simulink model "North_Country_Grid"  (R2025a)
settings: Solver=VariableStepAuto  StartTime=0.0  StopTime=10  RelTol=1e-3
PreLoadFcn:
  | Ts=50e-6;
InitFcn:
  | xInitial = WindFarmType4AverageModelInit;
  | Ts=50e-6;
undefined symbols (not defined in the file): D1, D11, Delta, DiscIntNeverNeededParam, find_system, Fnom_I, Fnom_R, Idc_nom, lagging, level, pulse, test_alpha, Vdc_nom, VLL_nom_I, VLL_nom_R
libraries: spsSecondOrderFilterLib x47, powerlib_extras x38, simulink x34, spsThreePhaseVIMeasurementLib x30, spsFirstOrderFilterLib x29, simulink_extras x26, spsabctodq0Lib x25, spsThreePhaseTransformerTwoWindingsLib x19, spsThreePhaseBreakerLib x18, spsThreePhasePISectionLineLib x17, spsControlledVoltageSourceLib x15, spsOnDelayLib x12
(part 10 of 18)

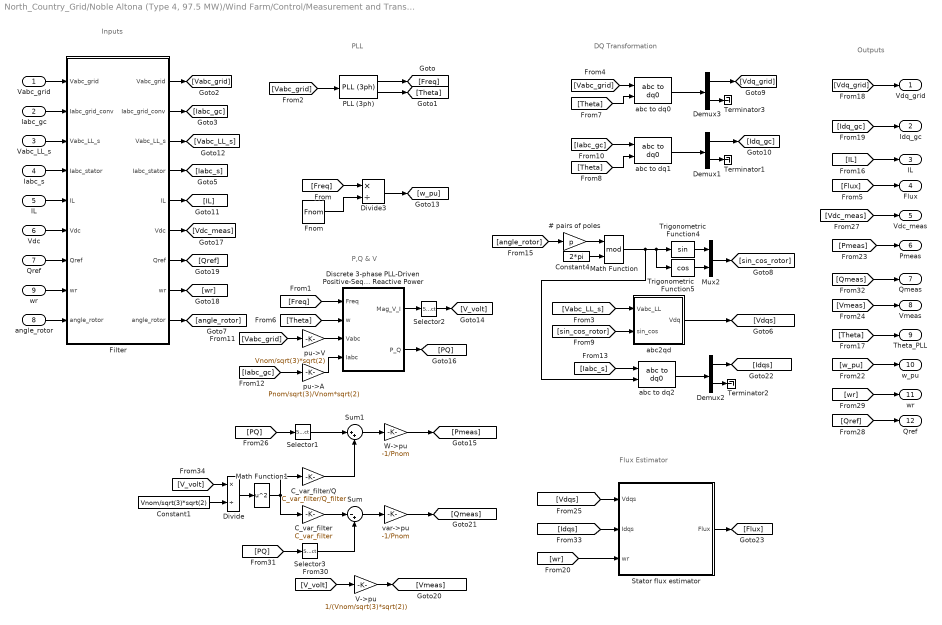
== system North_Country_Grid/Noble Altona (Type 4, 97.5 MW)/Wind Farm/Control/Measurement and Transformation ==
  note: Flux Estimator
  note: Outputs
  note: PLL
  note: DQ Transformation
  note: P,Q & V
  note: Inputs
  Vabc_grid : Inport
  Iabc_gc : Inport  Port=2
  Vabc_LL_s : Inport  Port=3
  Iabc_s : Inport  Port=4
  IL : Inport  Port=5
  Vdc : Inport  Port=6
  Qref : Inport  Port=7
  angle_rotor : Inport  Port=8
  wr : Inport  Port=9
  # pairs of poles : Gain  Gain=p  SaturateOnIntegerOverflow=on  OutDataTypeStr=Inherit: Same as input  ParamDataTypeStr=Inherit: Same as input
  C_var_filter : Gain  Gain=C_var_filter  SaturateOnIntegerOverflow=on  OutDataTypeStr=Inherit: Same as input  ParamDataTypeStr=Inherit: Same as input
  C_var_filter/Q : Gain  Gain=C_var_filter/Q_filter  SaturateOnIntegerOverflow=on  OutDataTypeStr=Inherit: Same as input  ParamDataTypeStr=Inherit: Same as input
  Constant1 : Constant  Value=Vnom/sqrt(3)*sqrt(2)
  Constant4 : Constant  Value=2*pi
  Demux1 : Demux  Outputs=[2 1]
      settings: DisplayOption=none
  Demux2 : Demux  Outputs=[2 1]
      settings: DisplayOption=none
  Demux3 : Demux  Outputs=[2 1]
      settings: DisplayOption=none
  Discrete 3-phase PLL-Driven Positive-Sequence Active & Reactive Power : Subsystem  mask(Discrete 3-phase PLL-Driven Positive-Sequence Active & Reactive Power){Finit=Fnom, Fmin=Fnom*45/60, Par_Vinit=[Vnom/sqrt(3)*sqrt(2) 30], Par_Iinit=[Pnom/sqrt(3)/Vnom*sqrt(2) -10], Ts=Ts}
      mask prompts: Finit "Initial frequency (Hz):"; Fmin "Minimum frequency (Hz):"; Par_Vinit "Voltage initial input: [ Mag  Phase(Degrees) ]"; Par_Iinit "Current initial input: [ Mag  Phase(Degrees) ]"; Ts "Sample time:"
      mask help:
      | This discrete block measures the 3-phase active power P and reactive power Q  associated with a periodic set of 3-phase voltages and currents which may contain harmonics. P and Q are calculated by evaluating the fundamental values (positive-sequence) of the input voltages and currents with a running window over one cycle of the specified frequency (port Freq).
      |  Input port "Sin_Cos" (a two-dimension signal) provides the reference frame required for the computation.
      |
      | input 1: must give the frequency of the fundamental (Hz)
      | Input 2: must contain a  [sin(wt)  cos(wt)] two dimension signal , where w is the rotation speed (rad/s) of the reference frame used for the computation..
      | input 3: Vectorized 3-phase  instantaneous voltage (Vabc)
      | input 4: Vectorized 3-phase instantaneous current (Iabc)
      |
      | Output 1: Vector [Mag_V Mag_I] of the fundamental values (Magnitude) of the voltage & current (peak values of the positive-sequence)
      | Output 2: 3-phase PQ measurement vector [P(W) Q (var)] evaluated at the specified frequency. Current flowing into an RL circuit will produce  positive active and reactive powers.
      |
      | For the first cycle of simulation, the outputs are held constant using the values specified by the parameters "Initial input".
      | he value of the parameter "Minimum frequency" is used to determine the buffer size of the "Variable Transport Delay" block found inside this subsystem.
      mask init:
      | power_initmask();
      settings: OpenFcn=power_openblockproxy();
  Divide : Product  Inputs=*/
  Divide3 : Product  Inputs=*/
  Filter : Subsystem  mask{Freq=Freq_filter, Zeta=Zeta_filter, Ts=Ts}
      mask prompts: Freq "Cut-off frequency (Hz):"; Zeta "Damping factor Zeta:"; Ts "Sample time"
  Fnom : Constant  Value=Fnom
  Math Function : Math  Operator=mod  SignedPower=on
  Math Function1 : Math  Operator=square  SignedPower=on
  Mux2 : Mux  Inputs=2
  PLL (3ph) : spsPLL3phLib/PLL (3ph)  Fmin=0.75*Fnom  Par_Init=[-45 Fnom]  ParK=[60 1400 1]  TcD=1e-4  MaxRateChangeFreq=12  FilterCutOffFreq=25  Ts=Ts  AGC=on
  Selector1 : Selector  InputPortWidth=2  IndexOptions=Index vector (dialog)  Indices=1  OutputSizes=1
  Selector2 : Selector  InputPortWidth=2  IndexOptions=Index vector (dialog)  Indices=1  OutputSizes=1
  Selector3 : Selector  InputPortWidth=2  IndexOptions=Index vector (dialog)  Indices=2  OutputSizes=1
  Stator flux estimator : Subsystem
  Sum : Sum  Inputs=|-+
  Sum1 : Sum  Inputs=|++
  Terminator1 : Terminator
  Terminator2 : Terminator
  Terminator3 : Terminator
  Trigonometric Function4 : Trigonometry
  Trigonometric Function5 : Trigonometry  Operator=cos
  V->pu : Gain  Gain=1/(Vnom/sqrt(3)*sqrt(2))  SaturateOnIntegerOverflow=on  OutDataTypeStr=Inherit: Same as input  ParamDataTypeStr=Inherit: Same as input
  W->pu : Gain  Gain=-1/Pnom  SaturateOnIntegerOverflow=on  OutDataTypeStr=Inherit: Same as input  ParamDataTypeStr=Inherit: Same as input
  abc to dq0 : spsabctodq0Lib/abc to dq0  Alignment=90 degrees behind phase A axis
  abc to dq1 : spsabctodq0Lib/abc to dq0  Alignment=90 degrees behind phase A axis
  abc to dq2 : spsabctodq0Lib/abc to dq0  Alignment=90 degrees behind phase A axis
  abc2qd : Subsystem
  pu->A : Gain  Gain=Pnom/sqrt(3)/Vnom*sqrt(2)  SaturateOnIntegerOverflow=on  OutDataTypeStr=Inherit: Same as input  ParamDataTypeStr=Inherit: Same as input
  pu->V : Gain  Gain=Vnom/sqrt(3)*sqrt(2)  SaturateOnIntegerOverflow=on  OutDataTypeStr=Inherit: Same as input  ParamDataTypeStr=Inherit: Same as input
  "var->pu " : Gain  Gain=-1/Pnom  SaturateOnIntegerOverflow=on  OutDataTypeStr=Inherit: Same as input  ParamDataTypeStr=Inherit: Same as input
  Vdq_grid : Outport  VectorParamsAs1DForOutWhenUnconnected=off
  Idq_gc : Outport  Port=2  VectorParamsAs1DForOutWhenUnconnected=off
  "IL " : Outport  Port=3  VectorParamsAs1DForOutWhenUnconnected=off
  Flux : Outport  Port=4  VectorParamsAs1DForOutWhenUnconnected=off
  Vdc_meas : Outport  Port=5  VectorParamsAs1DForOutWhenUnconnected=off
  Pmeas : Outport  Port=6  VectorParamsAs1DForOutWhenUnconnected=off
  Qmeas : Outport  Port=7  VectorParamsAs1DForOutWhenUnconnected=off
  Vmeas : Outport  Port=8  VectorParamsAs1DForOutWhenUnconnected=off
  Theta_PLL : Outport  Port=9  VectorParamsAs1DForOutWhenUnconnected=off
  w_pu : Outport  Port=10  VectorParamsAs1DForOutWhenUnconnected=off
  "wr " : Outport  Port=11  VectorParamsAs1DForOutWhenUnconnected=off
  "Qref " : Outport  Port=12  VectorParamsAs1DForOutWhenUnconnected=off
  wires:
  Filter/9("angle_rotor ") -> [angle_rotor]
  angle_rotor/1 -> Filter/9(angle_rotor)
  Stator flux estimator/1(Flux) -> [Flux]
  # pairs of poles/1 -> Math Function/1
  Constant4/1 -> Math Function/2
  abc2qd/1(Vdq) -> [Vdqs]
  Trigonometric Function5/1 -> Mux2/2
  Trigonometric Function4/1 -> Mux2/1
  [angle_rotor] -> # pairs of poles/1
  [Vabc_LL_s] -> abc2qd/1(Vabc_LL)
  [sin_cos_rotor] -> abc2qd/2(sin_cos)
  Mux2/1 -> [sin_cos_rotor]
  Demux2/1 -> [Idqs]
  Demux2/2 -> Terminator2/1
  abc to dq2/1 -> Demux2/1
  [Iabc_s] -> abc to dq2/1
  [Vdqs] -> Stator flux estimator/1(Vdqs)
  [Idqs] -> Stator flux estimator/2(Idqs)
  [wr] -> Stator flux estimator/3(wr)
  [Qmeas] -> Qmeas/1
  "var->pu "/1 -> [Qmeas]
  [PQ] -> Selector3/1
  V->pu/1 -> [Vmeas]
  [V_volt] -> V->pu/1
  Selector2/1 -> [V_volt]
  Discrete 3-phase PLL-Driven Positive-Sequence Active & Reactive Power/1(Mag_V_I) -> Selector2/1
  Demux1/2 -> Terminator1/1
  Demux3/1 -> [Vdq_grid]
  Demux3/2 -> Terminator3/1
  abc to dq1/1 -> Demux1/1
  abc to dq0/1 -> Demux3/1
  PLL (3ph)/1 -> [Freq]
  Fnom/1 -> Divide3/2
  Divide3/1 -> [w_pu]
  pu->V/1 -> Discrete 3-phase PLL-Driven Positive-Sequence Active & Reactive Power/3(Vabc)
  W->pu/1 -> [Pmeas]
  [Freq] -> Divide3/1
  [Freq] -> Discrete 3-phase PLL-Driven Positive-Sequence Active & Reactive Power/1(Freq)
  PLL (3ph)/2 -> [Theta]
  [Vabc_grid] -> abc to dq0/1
  [Theta] -> Discrete 3-phase PLL-Driven Positive-Sequence Active & Reactive Power/2(w)
  [Theta] -> abc to dq0/2
  [Theta] -> abc to dq1/2
  [Vabc_grid] -> PLL (3ph)/1
  [Iabc_gc] -> abc to dq1/1
  [Theta] -> Theta_PLL/1
  Demux1/1 -> [Idq_gc]
  [Vdq_grid] -> Vdq_grid/1
  [Idq_gc] -> Idq_gc/1
  [w_pu] -> w_pu/1
  [Pmeas] -> Pmeas/1
  [Vmeas] -> Vmeas/1
  pu->A/1 -> Discrete 3-phase PLL-Driven Positive-Sequence Active & Reactive Power/4(Iabc)
  [PQ] -> Selector1/1
  [Vdc_meas] -> Vdc_meas/1
  [Qref] -> "Qref "/1
  [wr] -> "wr "/1
  [Flux] -> Flux/1
  [Vabc_grid] -> pu->V/1
  [Iabc_gc] -> pu->A/1
  Discrete 3-phase PLL-Driven Positive-Sequence Active & Reactive Power/2(P_Q) -> [PQ]
  Vabc_grid/1 -> Filter/1(Vabc_grid)
  Vdc/1 -> Filter/6(Vdc)
  Qref/1 -> Filter/7(Qref)
  wr/1 -> Filter/8(wr)
  Filter/1("Vabc_grid ") -> [Vabc_grid]
  Filter/2("Iabc_grid_conv ") -> [Iabc_gc]
  Filter/4("Iabc_stator ") -> [Iabc_s]
  Filter/6("Vdc ") -> [Vdc_meas]
  Filter/8("wr ") -> [wr]
  Filter/7("Qref ") -> [Qref]
  Iabc_gc/1 -> Filter/2(Iabc_grid_conv)
  Iabc_s/1 -> Filter/4(Iabc_stator)
  Vabc_LL_s/1 -> Filter/3(Vabc_LL_s)
  Filter/3("Vabc_LL_s ") -> [Vabc_LL_s]
  [V_volt] -> Divide/1
  Constant1/1 -> Divide/2
  Divide/1 -> Math Function1/1
  Selector3/1 -> Sum/2
  C_var_filter/1 -> Sum/1
  Sum/1 -> "var->pu "/1
  Math Function1/1 -> C_var_filter/Q/1, C_var_filter/1
  Selector1/1 -> Sum1/1
  C_var_filter/Q/1 -> Sum1/2
  Sum1/1 -> W->pu/1
  IL/1 -> Filter/5(IL)
  Filter/5("IL ") -> [IL]
  [IL] -> "IL "/1
  Math Function/1 -> abc to dq2/2, Trigonometric Function5/1, Trigonometric Function4/1

== system North_Country_Grid/Noble Altona (Type 4, 97.5 MW)/Wind Farm/Control/Speed & Pitch Control ==
  note: Pitch Control
  note: Pitch Compensation
  note: Speed Regulator
  note: Note :
      | This control system is based on the report:
      | Dynamic Modeling of GE 1.5 and 3.6 Wind Turbine-Generators;
      | Prepared by: Nicholas W. Miller, William W. Price, Juan J. Sanchez-Gasca;
      | October 27, 2003, Version 3.0
      | GE-Power Systems Energy Consulting
      | Copyright 2002 General Electric Company, U.S.A.
      |
      | Another reference is:
      |
      | DYNAMIC MODELING OF GE 1.5 AND 3.6 MW WIND TURBINE GENERATORS
      | FOR STABILITY SIMULATIONS
      | Nicholas W. Miller, Juan J. Sanchez-Gasca, William W. Price Robert W. Delmerico
      | GE Power Systems GE Research
      | Schenectady, NY Niskayuna, NY
      |
      | 0-7803-7989-6/03/$17.00 02003 IEEE
  note: IL ref
  note: Current Regulator
  wr : Inport
  Pmeas : Inport  Port=2
  IL : Inport  Port=3
  0-inf : Saturate  UpperLimit=inf  LowerLimit=0
  0-pitch_max : Saturate  UpperLimit=pitch_max  LowerLimit=0
  "0-pitch_max " : Saturate  UpperLimit=pitch_max  LowerLimit=0
  Constant2 : Constant
  Discrete PI Controller : Subsystem  DialogController=POWERSYS.PowerSysDialog  mask(Discrete PI Controller){Kp=Kp_speed, Ki=Ki_speed, Par_Limits=[1.1 0], Init=0, Ts=Ts}
      mask prompts: Kp "Proportional gain (Kp):"; Ki "Integral gain (Ki):"; Par_Limits "Output limits: [ Upper   Lower ]"; Init "Output initial value:"; Ts "Sample time:"
      mask help: This block implements a discrete PI controller.
      mask init:
      | UpperLimit=Par_Limits(1);
      | LowerLimit=Par_Limits(2);
      | power_initmask();
      mask Help: This block is part of a subset of blocks in the Extras library that does not have documentation associated with it, other than the block mask description.
      mask Display: disp('PI');
  Discrete PI Controller1 : Subsystem  DialogController=POWERSYS.PowerSysDialog  mask(Discrete PI Controller){Kp=Kp_compensation, Ki=Ki_compensation, Par_Limits=[pitch_max 0], Init=0, Ts=Ts}
      mask prompts: Kp "Proportional gain (Kp):"; Ki "Integral gain (Ki):"; Par_Limits "Output limits: [ Upper   Lower ]"; Init "Output initial value:"; Ts "Sample time:"
      mask help: This block implements a discrete PI controller.
      mask init:
      | UpperLimit=Par_Limits(1);
      | LowerLimit=Par_Limits(2);
      | power_initmask();
      mask Help: This block is part of a subset of blocks in the Extras library that does not have documentation associated with it, other than the block mask description.
      mask Display: disp('PI');
  Discrete PI Controller2 : Subsystem  DialogController=POWERSYS.PowerSysDialog  mask(Discrete PI Controller){Kp=Kp_boost_cur_reg, Ki=Ki_boost_cur_reg, Par_Limits=[1 0], Init=0.5, Ts=Ts}
      mask prompts: Kp "Proportional gain (Kp):"; Ki "Integral gain (Ki):"; Par_Limits "Output limits: [ Upper   Lower ]"; Init "Output initial value:"; Ts "Sample time:"
      mask help: This block implements a discrete PI controller.
      mask init:
      | UpperLimit=Par_Limits(1);
      | LowerLimit=Par_Limits(2);
      | power_initmask();
      mask Help: This block is part of a subset of blocks in the Extras library that does not have documentation associated with it, other than the block mask description.
      mask Display: disp('PI');
  First-Order Filter : spsFirstOrderFilterLib/First-Order Filter  FilterType=Lowpass  Tc=Pitch_time_constant  Ts=Ts  Initialize=on  Vac_Init=[0.8 -25 60]*0  Vdc_Init=0  PlotResponse=off  FreqRange="[0,  200,  1]"
  First-Order Filter1 : spsFirstOrderFilterLib/First-Order Filter  FilterType=Lowpass  Tc=T_speed  Ts=Ts  Initialize=on  Vac_Init=[0, 0, 0]  Vdc_Init=1+init(1)/100  PlotResponse=off  FreqRange="[0,  200,  1]"
  Gain2 : Gain  Gain=Kp_pitch  SaturateOnIntegerOverflow=on  OutDataTypeStr=Inherit: Same as input  ParamDataTypeStr=Inherit: Same as input
  Rate Limiter   1 : RateLimiter  RisingSlewLimit=pitch_rate  FallingSlewLimit=-pitch_rate
  Sum : Sum  Inputs=-+  SaturateOnIntegerOverflow=on
  Sum1 : Sum  Inputs=|+-
  Sum2 : Sum  Inputs=|+-  SaturateOnIntegerOverflow=on
  Sum3 : Sum  Inputs=|++
  Sum4 : Sum  Inputs=|+-
  Switch : Switch  Threshold=0.75  SaturateOnIntegerOverflow=off  InputSameDT=off
  Tracking Curve : Fcn  Expr=-0.5551*u(1)^2+1.183*u(1)+0.425
  pu_elec->pu_mec : Gain  Gain=Pnom/Pmec
  wref : Constant
  Duty_Cycle : Outport  VectorParamsAs1DForOutWhenUnconnected=off
  Pitch (deg) : Outport  Port=2  VectorParamsAs1DForOutWhenUnconnected=off
  wires:
  wr/1 -> Sum/2, Sum1/1  "wr"
  0-inf/1 -> pu_elec->pu_mec/1
  pu_elec->pu_mec/1 -> Tracking Curve/1, Sum2/1, Switch/2  "Pmes"
  wref/1 -> Switch/1
  Switch/1 -> First-Order Filter1/1
  Sum1/1 -> Discrete PI Controller/1(Error)
  Constant2/1 -> Sum2/2  "Pref"
  Sum3/1 -> Rate Limiter   1/1
  Rate Limiter   1/1 -> "0-pitch_max "/1
  Gain2/1 -> 0-pitch_max/1
  Discrete PI Controller1/1(Out) -> Sum3/2  "Pitch_comp"
  Pmeas/1 -> 0-inf/1
  0-pitch_max/1 -> Sum3/1  "Pitch_contrl"
  "0-pitch_max "/1 -> First-Order Filter/1
  Sum/1 -> Gain2/1
  First-Order Filter/1 -> Pitch (deg)/1  "Pitch"
  Sum2/1 -> Discrete PI Controller1/1(Error)
  First-Order Filter1/1 -> Sum1/2, Sum/1  "wref"
  Tracking Curve/1 -> Switch/3
  Discrete PI Controller/1(Out) -> Sum4/1
  Sum4/1 -> Discrete PI Controller2/1(Error)
  IL/1 -> Sum4/2
  Discrete PI Controller2/1(Out) -> Duty_Cycle/1  "Duty cycle"

== system North_Country_Grid/Noble Chateauguay (Type 4, 106.5 MW)/Wind Farm/Control/Excitation Control system ==
  Flux : Inport
  wr : Inport  Port=2
  Discrete PI Controller : Subsystem  DialogController=POWERSYS.PowerSysDialog  mask(Discrete PI Controller){Kp=Kp_field, Ki=Ki_field, Par_Limits=[1 0]*Vf_limit, Init=init(9), Ts=Ts}
      mask prompts: Kp "Proportional gain (Kp):"; Ki "Integral gain (Ki):"; Par_Limits "Output limits: [ Upper   Lower ]"; Init "Output initial value:"; Ts "Sample time:"
      mask help: This block implements a discrete PI controller.
      mask init:
      | UpperLimit=Par_Limits(1);
      | LowerLimit=Par_Limits(2);
      | power_initmask();
      mask Help: This block is part of a subset of blocks in the Extras library that does not have documentation associated with it, other than the block mask description.
      mask Display: disp('PI');
  Divide : Product  Inputs=*/
  Flux_ref : Constant
  "Flux_ref " : Constant
  Sum4 : Sum  Inputs=|+-  InputSameDT=on  SaturateOnIntegerOverflow=on  OutDataTypeStr=Inherit: Same as first input
  Switch : Switch  Threshold=1  SaturateOnIntegerOverflow=off  InputSameDT=off
  avoid division by 0 : Saturate  UpperLimit=inf  LowerLimit=1e-6
  Vf : Outport  VectorParamsAs1DForOutWhenUnconnected=off
  wires:
  Sum4/1 -> Discrete PI Controller/1(Error)
  Discrete PI Controller/1(Out) -> Vf/1  "Vf"
  Flux/1 -> Sum4/2  "Flux"
  wr/1 -> Switch/2, avoid division by 0/1
  Flux_ref/1 -> Switch/3
  "Flux_ref "/1 -> Divide/1
  avoid division by 0/1 -> Divide/2
  Divide/1 -> Switch/1
  Switch/1 -> Sum4/1

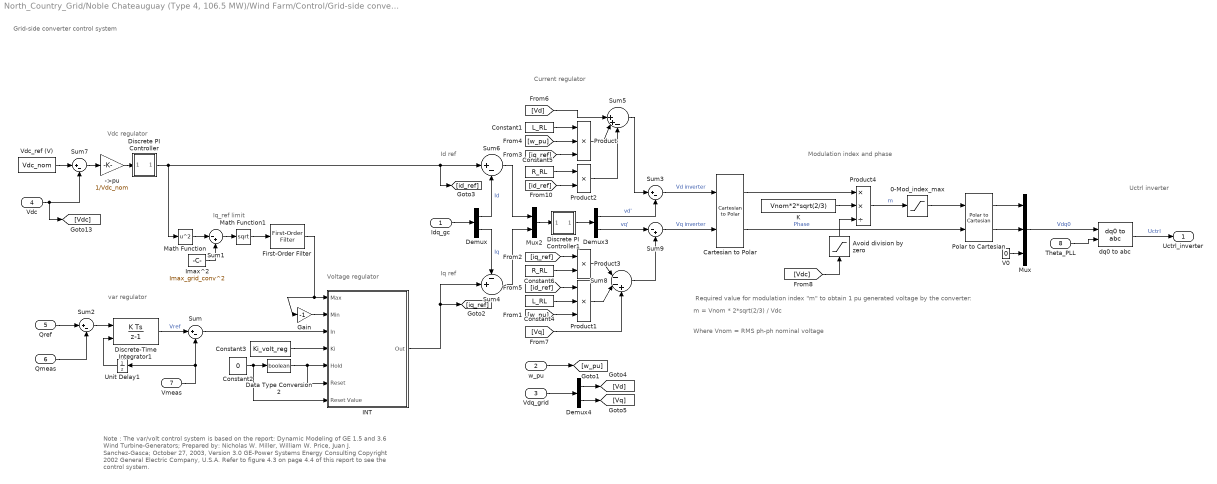
== system North_Country_Grid/Noble Chateauguay (Type 4, 106.5 MW)/Wind Farm/Control/Grid-side converter Control system ==
  note: Grid-side converter control system
  note: var regulator
  note: Voltage regulator
  note: Vdc regulator
  note: Iq_ref limit
  note: Current regulator
  note: Id ref
  note: Iq ref
  note: Required value for modulation index "m" to obtain 1 pu generated voltage by the converter:
  note: m = Vnom * 2*sqrt(2/3) / Vdc
  note: Where Vnom = RMS ph-ph nominal voltage
  note: Modulation index and phase
  note: Uctrl inverter
  note: Note :
      | The var/volt control system is based on the report:
      | Dynamic Modeling of GE 1.5 and 3.6 Wind Turbine-Generators;
      | Prepared by: Nicholas W. Miller, William W. Price, Juan J. Sanchez-Gasca;
      | October 27, 2003, Version 3.0
      | GE-Power Systems Energy Consulting
      | Copyright 2002 General Electric Company, U.S.A.
      |
      | Refer to figure 4.3 on page 4.4 of this report to see the control system.
  Idq_gc : Inport
  w_pu : Inport  Port=2
  Vdq_grid : Inport  Port=3
  Vdc : Inport  Port=4
  Qref : Inport  Port=5
  Qmeas : Inport  Port=6
  Vmeas : Inport  Port=7
  Theta_PLL : Inport  Port=8
  ->pu : Gain  Gain=1/Vdc_nom
  0-Mod_index_max : Saturate  UpperLimit=Mod_index_max  LowerLimit=0
  Avoid division by zero : Saturate  UpperLimit=1e6  LowerLimit=1e-6
  Cartesian to Polar : simulink_extras/Transformations/Cartesian to Polar
  Constant1 : Constant  Value=L_RL
  Constant2 : Constant  Value=0
  Constant3 : Constant  Value=Ki_volt_reg
  Constant4 : Constant  Value=L_RL
  Constant5 : Constant  Value=R_RL
  Constant6 : Constant  Value=R_RL
  Data Type Conversion2 : DataTypeConversion  OutDataTypeStr=boolean  SaturateOnIntegerOverflow=off  RndMeth=Floor
  Demux : Demux  Outputs=2
      settings: DisplayOption=none
  Demux3 : Demux  Outputs=2
      settings: DisplayOption=none
  Demux4 : Demux  Outputs=2
      settings: DisplayOption=none
  Discrete PI Controller : Subsystem  DialogController=POWERSYS.PowerSysDialog  mask(Discrete PI Controller){Kp=Kp_dc, Ki=Ki_dc, Par_Limits=[1 -1]*Imax_grid_conv, Init=0, Ts=Ts}
      mask prompts: Kp "Proportional gain (Kp):"; Ki "Integral gain (Ki):"; Par_Limits "Output limits: [ Upper   Lower ]"; Init "Output initial value:"; Ts "Sample time:"
      mask help: This block implements a discrete PI controller.
      mask init:
      | UpperLimit=Par_Limits(1);
      | LowerLimit=Par_Limits(2);
      | power_initmask();
      mask Help: This block is part of a subset of blocks in the Extras library that does not have documentation associated with it, other than the block mask description.
      mask Display: disp('PI');
  Discrete PI Controller1 : Subsystem  DialogController=POWERSYS.PowerSysDialog  mask(Discrete PI Controller){Kp=Kp_grid_side_cur_reg, Ki=Ki_grid_side_cur_reg, Par_Limits=[1 -1]*Current_reg_output_limit, Init=0, Ts=Ts}
      mask prompts: Kp "Proportional gain (Kp):"; Ki "Integral gain (Ki):"; Par_Limits "Output limits: [ Upper   Lower ]"; Init "Output initial value:"; Ts "Sample time:"
      mask help: This block implements a discrete PI controller.
      mask init:
      | UpperLimit=Par_Limits(1);
      | LowerLimit=Par_Limits(2);
      | power_initmask();
      mask Help: This block is part of a subset of blocks in the Extras library that does not have documentation associated with it, other than the block mask description.
      mask Display: disp('PI');
  Discrete-Time Integrator1 : DiscreteIntegrator  gainval=Ki_var_reg  InitialConditionSource=external  InitialCondition=1  SampleTime=Ts  LimitOutput=on  UpperSaturationLimit=Var_reg_output_hi_limit  LowerSaturationLimit=Var_reg_output_low_limit  ICPrevOutput=DiscIntNeverNeededParam  ICPrevScaledInput=DiscIntNeverNeededParam
  First-Order Filter : spsFirstOrderFilterLib/First-Order Filter  FilterType=Lowpass  Tc=Iq_ref_limit_time_constant  Ts=Ts  Initialize=on  Vac_Init=[0, 0, 0]  Vdc_Init=Imax_grid_conv  PlotResponse=off  FreqRange="[0,  200,  1]"
  Gain : Gain  Gain=-1  SaturateOnIntegerOverflow=on  OutDataTypeStr=Inherit: Same as input  ParamDataTypeStr=Inherit: Same as input
  INT : Subsystem  mask(Integrator  With  External  Dynamic  Limits (Discrete)){}
      mask Display: disp('Discrete-Time\n(Trapezoidal)\nIntegrator\n ')
  Imax^2 : Constant  Value=Imax_grid_conv^2
  K : Constant  Value=Vnom*2*sqrt(2/3)
  Math Function : Math  Operator=square  SignedPower=on
  Math Function1 : Math  Operator=sqrt  SignedPower=on
  Mux : Mux  Inputs=3
  Mux2 : Mux  Inputs=2
  Polar to Cartesian : simulink_extras/Transformations/Polar to Cartesian
  Product : Product  Inputs=3  InputSameDT=on  SaturateOnIntegerOverflow=on  OutDataTypeStr=Inherit: Same as first input
  Product1 : Product  Inputs=3  InputSameDT=on  SaturateOnIntegerOverflow=on  OutDataTypeStr=Inherit: Same as first input
  Product2 : Product  InputSameDT=on  SaturateOnIntegerOverflow=on  OutDataTypeStr=Inherit: Same as first input
  Product3 : Product  InputSameDT=on  SaturateOnIntegerOverflow=on  OutDataTypeStr=Inherit: Same as first input
  Product4 : Product  Inputs=**/  InputSameDT=on  SaturateOnIntegerOverflow=on  OutDataTypeStr=Inherit: Same as first input
  Sum{,2..3,6..7} (5 alike) : Sum  Inputs=|+-  InputSameDT=on  SaturateOnIntegerOverflow=on  OutDataTypeStr=Inherit: Same as first input
  Sum1 : Sum  Inputs=|-+  InputSameDT=on  SaturateOnIntegerOverflow=on  OutDataTypeStr=Inherit: Same as first input
  Sum4 : Sum  Inputs=-+|  InputSameDT=on  SaturateOnIntegerOverflow=on  OutDataTypeStr=Inherit: Same as first input
  Sum5 : Sum  Inputs=||++-  InputSameDT=on  SaturateOnIntegerOverflow=on  OutDataTypeStr=Inherit: Same as first input
  Sum8 : Sum  Inputs=|--+  InputSameDT=on  SaturateOnIntegerOverflow=on  OutDataTypeStr=Inherit: Same as first input
  Sum9 : Sum  Inputs=|-+  InputSameDT=on  SaturateOnIntegerOverflow=on  OutDataTypeStr=Inherit: Same as first input
  Unit Delay1 : UnitDelay  InitialCondition=1  SampleTime=Ts  HasFrameUpgradeWarning=on
  V0 : Constant  Value=0
  Vdc_ref (V) : Constant  Value=Vdc_nom
  dq0 to abc : spsdq0toabcLib/dq0 to abc  Alignment=90 degrees behind phase A axis
  Uctrl_inverter : Outport  VectorParamsAs1DForOutWhenUnconnected=off
  wires:
  Vdc/1 -> [Vdc], Sum7/2
  Vdq_grid/1 -> Demux4/1
  Sum7/1 -> ->pu/1
  ->pu/1 -> Discrete PI Controller/1(Error)
  Discrete PI Controller/1(Out) -> Math Function/1, [id_ref], Sum6/1
  Sum/1 -> INT/3(In)
  Constant2/1 -> Data Type Conversion2/1, INT/7(Reset Value)
  Data Type Conversion2/1 -> INT/5(Hold), INT/6(Reset)
  Gain/1 -> INT/2(Min)
  Constant3/1 -> INT/4(Ki)
  Discrete-Time Integrator1/1 -> Sum/1  "Vref"
  Vmeas/1 -> Unit Delay1/1, Sum/2
  Qmeas/1 -> Sum2/2
  Sum2/1 -> Discrete-Time Integrator1/1
  Unit Delay1/1 -> Discrete-Time Integrator1/2
  Math Function1/1 -> First-Order Filter/1
  Sum1/1 -> Math Function1/1
  Imax^2/1 -> Sum1/2
  Math Function/1 -> Sum1/1
  First-Order Filter/1 -> Gain/1, INT/1(Max)
  Constant4/1 -> Product1/2
  Discrete PI Controller1/1(Out) -> Demux3/1
  Mux2/1 -> Discrete PI Controller1/1(Error)
  Constant1/1 -> Product/1
  Demux/2 -> Sum4/1  "Iq"
  Demux/1 -> Sum6/2  "Id"
  Product/1 -> Sum5/2
  Constant5/1 -> Product2/1
  Constant6/1 -> Product3/2
  Product1/1 -> Sum8/2
  Product2/1 -> Sum5/3
  Product3/1 -> Sum8/1
  Sum6/1 -> Mux2/1
  Sum4/1 -> Mux2/2
  [w_pu] -> Product1/3
  [w_pu] -> Product/2
  [iq_ref] -> Product/3
  [id_ref] -> Product2/2
  [iq_ref] -> Product3/1
  [id_ref] -> Product1/1
  Demux3/1 -> Sum3/2  "vd'"
  Demux3/2 -> Sum9/1  "vq'"
  w_pu/1 -> [w_pu]
  Demux4/1 -> [Vd]
  Demux4/2 -> [Vq]
  [Vq] -> Sum8/3
  [Vd] -> Sum5/1
  Product4/1 -> 0-Mod_index_max/1  "m"
  K/1 -> Product4/2
  Avoid division by zero/1 -> Product4/3
  Cartesian to Polar/1 -> Product4/1
  [Vdc] -> Avoid division by zero/1
  Sum3/1 -> Cartesian to Polar/1  "Vd inverter"
  Sum9/1 -> Cartesian to Polar/2  "Vq inverter"
  Polar to Cartesian/2 -> Mux/2
  Polar to Cartesian/1 -> Mux/1
  V0/1 -> Mux/3
  Cartesian to Polar/2 -> Polar to Cartesian/2  "Phase"
  Mux/1 -> dq0 to abc/1  "Vdq0"
  dq0 to abc/1 -> Uctrl_inverter/1  "Uctrl"
  Idq_gc/1 -> Demux/1
  0-Mod_index_max/1 -> Polar to Cartesian/1
  Sum5/1 -> Sum3/1
  Sum8/1 -> Sum9/2
  Vdc_ref (V)/1 -> Sum7/1
  Qref/1 -> Sum2/1
  INT/1(Out) -> Sum4/2, [iq_ref]
  Theta_PLL/1 -> dq0 to abc/2

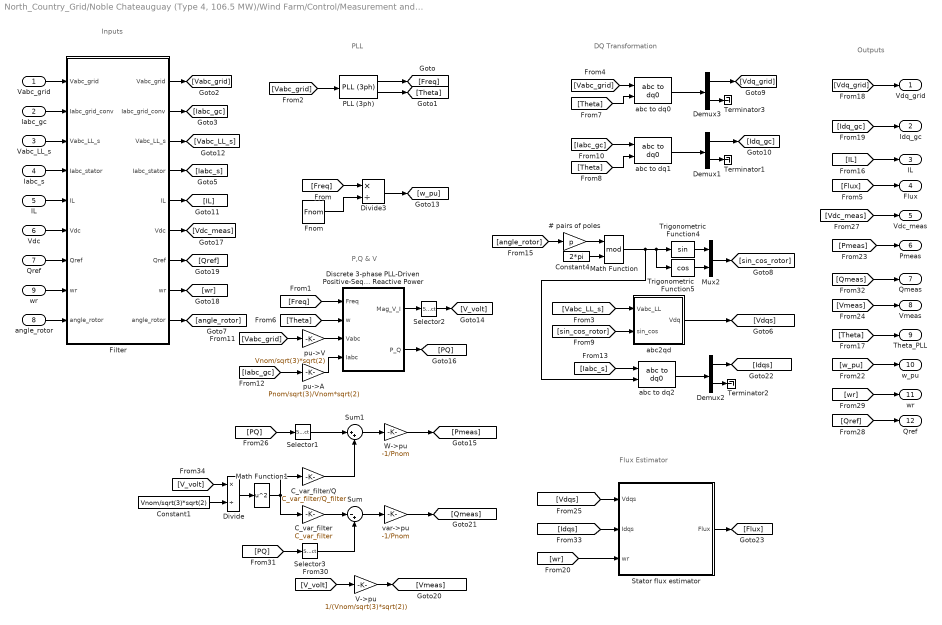
== system North_Country_Grid/Noble Chateauguay (Type 4, 106.5 MW)/Wind Farm/Control/Measurement and Transformation ==
  note: Flux Estimator
  note: Outputs
  note: PLL
  note: DQ Transformation
  note: P,Q & V
  note: Inputs
  Vabc_grid : Inport
  Iabc_gc : Inport  Port=2
  Vabc_LL_s : Inport  Port=3
  Iabc_s : Inport  Port=4
  IL : Inport  Port=5
  Vdc : Inport  Port=6
  Qref : Inport  Port=7
  angle_rotor : Inport  Port=8
  wr : Inport  Port=9
  # pairs of poles : Gain  Gain=p  SaturateOnIntegerOverflow=on  OutDataTypeStr=Inherit: Same as input  ParamDataTypeStr=Inherit: Same as input
  C_var_filter : Gain  Gain=C_var_filter  SaturateOnIntegerOverflow=on  OutDataTypeStr=Inherit: Same as input  ParamDataTypeStr=Inherit: Same as input
  C_var_filter/Q : Gain  Gain=C_var_filter/Q_filter  SaturateOnIntegerOverflow=on  OutDataTypeStr=Inherit: Same as input  ParamDataTypeStr=Inherit: Same as input
  Constant1 : Constant  Value=Vnom/sqrt(3)*sqrt(2)
  Constant4 : Constant  Value=2*pi
  Demux1 : Demux  Outputs=[2 1]
      settings: DisplayOption=none
  Demux2 : Demux  Outputs=[2 1]
      settings: DisplayOption=none
  Demux3 : Demux  Outputs=[2 1]
      settings: DisplayOption=none
  Discrete 3-phase PLL-Driven Positive-Sequence Active & Reactive Power : Subsystem  mask(Discrete 3-phase PLL-Driven Positive-Sequence Active & Reactive Power){Finit=Fnom, Fmin=Fnom*45/60, Par_Vinit=[Vnom/sqrt(3)*sqrt(2) 30], Par_Iinit=[Pnom/sqrt(3)/Vnom*sqrt(2) -10], Ts=Ts}
      mask prompts: Finit "Initial frequency (Hz):"; Fmin "Minimum frequency (Hz):"; Par_Vinit "Voltage initial input: [ Mag  Phase(Degrees) ]"; Par_Iinit "Current initial input: [ Mag  Phase(Degrees) ]"; Ts "Sample time:"
      mask help:
      | This discrete block measures the 3-phase active power P and reactive power Q  associated with a periodic set of 3-phase voltages and currents which may contain harmonics. P and Q are calculated by evaluating the fundamental values (positive-sequence) of the input voltages and currents with a running window over one cycle of the specified frequency (port Freq).
      |  Input port "Sin_Cos" (a two-dimension signal) provides the reference frame required for the computation.
      |
      | input 1: must give the frequency of the fundamental (Hz)
      | Input 2: must contain a  [sin(wt)  cos(wt)] two dimension signal , where w is the rotation speed (rad/s) of the reference frame used for the computation..
      | input 3: Vectorized 3-phase  instantaneous voltage (Vabc)
      | input 4: Vectorized 3-phase instantaneous current (Iabc)
      |
      | Output 1: Vector [Mag_V Mag_I] of the fundamental values (Magnitude) of the voltage & current (peak values of the positive-sequence)
      | Output 2: 3-phase PQ measurement vector [P(W) Q (var)] evaluated at the specified frequency. Current flowing into an RL circuit will produce  positive active and reactive powers.
      |
      | For the first cycle of simulation, the outputs are held constant using the values specified by the parameters "Initial input".
      | he value of the parameter "Minimum frequency" is used to determine the buffer size of the "Variable Transport Delay" block found inside this subsystem.
      mask init:
      | power_initmask();
      settings: OpenFcn=power_openblockproxy();
  Divide : Product  Inputs=*/
  Divide3 : Product  Inputs=*/
  Filter : Subsystem  mask{Freq=Freq_filter, Zeta=Zeta_filter, Ts=Ts}
      mask prompts: Freq "Cut-off frequency (Hz):"; Zeta "Damping factor Zeta:"; Ts "Sample time"
  Fnom : Constant  Value=Fnom
  Math Function : Math  Operator=mod  SignedPower=on
  Math Function1 : Math  Operator=square  SignedPower=on
  Mux2 : Mux  Inputs=2
  PLL (3ph) : spsPLL3phLib/PLL (3ph)  Fmin=0.75*Fnom  Par_Init=[-45 Fnom]  ParK=[60 1400 1]  TcD=1e-4  MaxRateChangeFreq=12  FilterCutOffFreq=25  Ts=Ts  AGC=on
  Selector1 : Selector  InputPortWidth=2  IndexOptions=Index vector (dialog)  Indices=1  OutputSizes=1
  Selector2 : Selector  InputPortWidth=2  IndexOptions=Index vector (dialog)  Indices=1  OutputSizes=1
  Selector3 : Selector  InputPortWidth=2  IndexOptions=Index vector (dialog)  Indices=2  OutputSizes=1
  Stator flux estimator : Subsystem
  Sum : Sum  Inputs=|-+
  Sum1 : Sum  Inputs=|++
  Terminator1 : Terminator
  Terminator2 : Terminator
  Terminator3 : Terminator
  Trigonometric Function4 : Trigonometry
  Trigonometric Function5 : Trigonometry  Operator=cos
  V->pu : Gain  Gain=1/(Vnom/sqrt(3)*sqrt(2))  SaturateOnIntegerOverflow=on  OutDataTypeStr=Inherit: Same as input  ParamDataTypeStr=Inherit: Same as input
  W->pu : Gain  Gain=-1/Pnom  SaturateOnIntegerOverflow=on  OutDataTypeStr=Inherit: Same as input  ParamDataTypeStr=Inherit: Same as input
  abc to dq0 : spsabctodq0Lib/abc to dq0  Alignment=90 degrees behind phase A axis
  abc to dq1 : spsabctodq0Lib/abc to dq0  Alignment=90 degrees behind phase A axis
  abc to dq2 : spsabctodq0Lib/abc to dq0  Alignment=90 degrees behind phase A axis
  abc2qd : Subsystem
  pu->A : Gain  Gain=Pnom/sqrt(3)/Vnom*sqrt(2)  SaturateOnIntegerOverflow=on  OutDataTypeStr=Inherit: Same as input  ParamDataTypeStr=Inherit: Same as input
  pu->V : Gain  Gain=Vnom/sqrt(3)*sqrt(2)  SaturateOnIntegerOverflow=on  OutDataTypeStr=Inherit: Same as input  ParamDataTypeStr=Inherit: Same as input
  "var->pu " : Gain  Gain=-1/Pnom  SaturateOnIntegerOverflow=on  OutDataTypeStr=Inherit: Same as input  ParamDataTypeStr=Inherit: Same as input
  Vdq_grid : Outport  VectorParamsAs1DForOutWhenUnconnected=off
  Idq_gc : Outport  Port=2  VectorParamsAs1DForOutWhenUnconnected=off
  "IL " : Outport  Port=3  VectorParamsAs1DForOutWhenUnconnected=off
  Flux : Outport  Port=4  VectorParamsAs1DForOutWhenUnconnected=off
  Vdc_meas : Outport  Port=5  VectorParamsAs1DForOutWhenUnconnected=off
  Pmeas : Outport  Port=6  VectorParamsAs1DForOutWhenUnconnected=off
  Qmeas : Outport  Port=7  VectorParamsAs1DForOutWhenUnconnected=off
  Vmeas : Outport  Port=8  VectorParamsAs1DForOutWhenUnconnected=off
  Theta_PLL : Outport  Port=9  VectorParamsAs1DForOutWhenUnconnected=off
  w_pu : Outport  Port=10  VectorParamsAs1DForOutWhenUnconnected=off
  "wr " : Outport  Port=11  VectorParamsAs1DForOutWhenUnconnected=off
  "Qref " : Outport  Port=12  VectorParamsAs1DForOutWhenUnconnected=off
  wires:
  Filter/9("angle_rotor ") -> [angle_rotor]
  angle_rotor/1 -> Filter/9(angle_rotor)
  Stator flux estimator/1(Flux) -> [Flux]
  # pairs of poles/1 -> Math Function/1
  Constant4/1 -> Math Function/2
  abc2qd/1(Vdq) -> [Vdqs]
  Trigonometric Function5/1 -> Mux2/2
  Trigonometric Function4/1 -> Mux2/1
  [angle_rotor] -> # pairs of poles/1
  [Vabc_LL_s] -> abc2qd/1(Vabc_LL)
  [sin_cos_rotor] -> abc2qd/2(sin_cos)
  Mux2/1 -> [sin_cos_rotor]
  Demux2/1 -> [Idqs]
  Demux2/2 -> Terminator2/1
  abc to dq2/1 -> Demux2/1
  [Iabc_s] -> abc to dq2/1
  [Vdqs] -> Stator flux estimator/1(Vdqs)
  [Idqs] -> Stator flux estimator/2(Idqs)
  [wr] -> Stator flux estimator/3(wr)
  [Qmeas] -> Qmeas/1
  "var->pu "/1 -> [Qmeas]
  [PQ] -> Selector3/1
  V->pu/1 -> [Vmeas]
  [V_volt] -> V->pu/1
  Selector2/1 -> [V_volt]
  Discrete 3-phase PLL-Driven Positive-Sequence Active & Reactive Power/1(Mag_V_I) -> Selector2/1
  Demux1/2 -> Terminator1/1
  Demux3/1 -> [Vdq_grid]
  Demux3/2 -> Terminator3/1
  abc to dq1/1 -> Demux1/1
  abc to dq0/1 -> Demux3/1
  PLL (3ph)/1 -> [Freq]
  Fnom/1 -> Divide3/2
  Divide3/1 -> [w_pu]
  pu->V/1 -> Discrete 3-phase PLL-Driven Positive-Sequence Active & Reactive Power/3(Vabc)
  W->pu/1 -> [Pmeas]
  [Freq] -> Divide3/1
  [Freq] -> Discrete 3-phase PLL-Driven Positive-Sequence Active & Reactive Power/1(Freq)
  PLL (3ph)/2 -> [Theta]
  [Vabc_grid] -> abc to dq0/1
  [Theta] -> Discrete 3-phase PLL-Driven Positive-Sequence Active & Reactive Power/2(w)
  [Theta] -> abc to dq0/2
  [Theta] -> abc to dq1/2
  [Vabc_grid] -> PLL (3ph)/1
  [Iabc_gc] -> abc to dq1/1
  [Theta] -> Theta_PLL/1
  Demux1/1 -> [Idq_gc]
  [Vdq_grid] -> Vdq_grid/1
  [Idq_gc] -> Idq_gc/1
  [w_pu] -> w_pu/1
  [Pmeas] -> Pmeas/1
  [Vmeas] -> Vmeas/1
  pu->A/1 -> Discrete 3-phase PLL-Driven Positive-Sequence Active & Reactive Power/4(Iabc)
  [PQ] -> Selector1/1
  [Vdc_meas] -> Vdc_meas/1
  [Qref] -> "Qref "/1
  [wr] -> "wr "/1
  [Flux] -> Flux/1
  [Vabc_grid] -> pu->V/1
  [Iabc_gc] -> pu->A/1
  Discrete 3-phase PLL-Driven Positive-Sequence Active & Reactive Power/2(P_Q) -> [PQ]
  Vabc_grid/1 -> Filter/1(Vabc_grid)
  Vdc/1 -> Filter/6(Vdc)
  Qref/1 -> Filter/7(Qref)
  wr/1 -> Filter/8(wr)
  Filter/1("Vabc_grid ") -> [Vabc_grid]
  Filter/2("Iabc_grid_conv ") -> [Iabc_gc]
  Filter/4("Iabc_stator ") -> [Iabc_s]
  Filter/6("Vdc ") -> [Vdc_meas]
  Filter/8("wr ") -> [wr]
  Filter/7("Qref ") -> [Qref]
  Iabc_gc/1 -> Filter/2(Iabc_grid_conv)
  Iabc_s/1 -> Filter/4(Iabc_stator)
  Vabc_LL_s/1 -> Filter/3(Vabc_LL_s)
  Filter/3("Vabc_LL_s ") -> [Vabc_LL_s]
  [V_volt] -> Divide/1
  Constant1/1 -> Divide/2
  Divide/1 -> Math Function1/1
  Selector3/1 -> Sum/2
  C_var_filter/1 -> Sum/1
  Sum/1 -> "var->pu "/1
  Math Function1/1 -> C_var_filter/Q/1, C_var_filter/1
  Selector1/1 -> Sum1/1
  C_var_filter/Q/1 -> Sum1/2
  Sum1/1 -> W->pu/1
  IL/1 -> Filter/5(IL)
  Filter/5("IL ") -> [IL]
  [IL] -> "IL "/1
  Math Function/1 -> abc to dq2/2, Trigonometric Function5/1, Trigonometric Function4/1

== system North_Country_Grid/Noble Chateauguay (Type 4, 106.5 MW)/Wind Farm/Control/Speed & Pitch Control ==
  note: Pitch Control
  note: Pitch Compensation
  note: Speed Regulator
  note: Note :
      | This control system is based on the report:
      | Dynamic Modeling of GE 1.5 and 3.6 Wind Turbine-Generators;
      | Prepared by: Nicholas W. Miller, William W. Price, Juan J. Sanchez-Gasca;
      | October 27, 2003, Version 3.0
      | GE-Power Systems Energy Consulting
      | Copyright 2002 General Electric Company, U.S.A.
      |
      | Another reference is:
      |
      | DYNAMIC MODELING OF GE 1.5 AND 3.6 MW WIND TURBINE GENERATORS
      | FOR STABILITY SIMULATIONS
      | Nicholas W. Miller, Juan J. Sanchez-Gasca, William W. Price Robert W. Delmerico
      | GE Power Systems GE Research
      | Schenectady, NY Niskayuna, NY
      |
      | 0-7803-7989-6/03/$17.00 02003 IEEE
  note: IL ref
  note: Current Regulator
  wr : Inport
  Pmeas : Inport  Port=2
  IL : Inport  Port=3
  0-inf : Saturate  UpperLimit=inf  LowerLimit=0
  0-pitch_max : Saturate  UpperLimit=pitch_max  LowerLimit=0
  "0-pitch_max " : Saturate  UpperLimit=pitch_max  LowerLimit=0
  Constant2 : Constant
  Discrete PI Controller : Subsystem  DialogController=POWERSYS.PowerSysDialog  mask(Discrete PI Controller){Kp=Kp_speed, Ki=Ki_speed, Par_Limits=[1.1 0], Init=0, Ts=Ts}
      mask prompts: Kp "Proportional gain (Kp):"; Ki "Integral gain (Ki):"; Par_Limits "Output limits: [ Upper   Lower ]"; Init "Output initial value:"; Ts "Sample time:"
      mask help: This block implements a discrete PI controller.
      mask init:
      | UpperLimit=Par_Limits(1);
      | LowerLimit=Par_Limits(2);
      | power_initmask();
      mask Help: This block is part of a subset of blocks in the Extras library that does not have documentation associated with it, other than the block mask description.
      mask Display: disp('PI');
  Discrete PI Controller1 : Subsystem  DialogController=POWERSYS.PowerSysDialog  mask(Discrete PI Controller){Kp=Kp_compensation, Ki=Ki_compensation, Par_Limits=[pitch_max 0], Init=0, Ts=Ts}
      mask prompts: Kp "Proportional gain (Kp):"; Ki "Integral gain (Ki):"; Par_Limits "Output limits: [ Upper   Lower ]"; Init "Output initial value:"; Ts "Sample time:"
      mask help: This block implements a discrete PI controller.
      mask init:
      | UpperLimit=Par_Limits(1);
      | LowerLimit=Par_Limits(2);
      | power_initmask();
      mask Help: This block is part of a subset of blocks in the Extras library that does not have documentation associated with it, other than the block mask description.
      mask Display: disp('PI');
  Discrete PI Controller2 : Subsystem  DialogController=POWERSYS.PowerSysDialog  mask(Discrete PI Controller){Kp=Kp_boost_cur_reg, Ki=Ki_boost_cur_reg, Par_Limits=[1 0], Init=0.5, Ts=Ts}
      mask prompts: Kp "Proportional gain (Kp):"; Ki "Integral gain (Ki):"; Par_Limits "Output limits: [ Upper   Lower ]"; Init "Output initial value:"; Ts "Sample time:"
      mask help: This block implements a discrete PI controller.
      mask init:
      | UpperLimit=Par_Limits(1);
      | LowerLimit=Par_Limits(2);
      | power_initmask();
      mask Help: This block is part of a subset of blocks in the Extras library that does not have documentation associated with it, other than the block mask description.
      mask Display: disp('PI');
  First-Order Filter : spsFirstOrderFilterLib/First-Order Filter  FilterType=Lowpass  Tc=Pitch_time_constant  Ts=Ts  Initialize=on  Vac_Init=[0.8 -25 60]*0  Vdc_Init=0  PlotResponse=off  FreqRange="[0,  200,  1]"
  First-Order Filter1 : spsFirstOrderFilterLib/First-Order Filter  FilterType=Lowpass  Tc=T_speed  Ts=Ts  Initialize=on  Vac_Init=[0, 0, 0]  Vdc_Init=1+init(1)/100  PlotResponse=off  FreqRange="[0,  200,  1]"
  Gain2 : Gain  Gain=Kp_pitch  SaturateOnIntegerOverflow=on  OutDataTypeStr=Inherit: Same as input  ParamDataTypeStr=Inherit: Same as input
  Rate Limiter   1 : RateLimiter  RisingSlewLimit=pitch_rate  FallingSlewLimit=-pitch_rate
  Sum : Sum  Inputs=-+  SaturateOnIntegerOverflow=on
  Sum1 : Sum  Inputs=|+-
  Sum2 : Sum  Inputs=|+-  SaturateOnIntegerOverflow=on
  Sum3 : Sum  Inputs=|++
  Sum4 : Sum  Inputs=|+-
  Switch : Switch  Threshold=0.75  SaturateOnIntegerOverflow=off  InputSameDT=off
  Tracking Curve : Fcn  Expr=-0.5551*u(1)^2+1.183*u(1)+0.425
  pu_elec->pu_mec : Gain  Gain=Pnom/Pmec
  wref : Constant
  Duty_Cycle : Outport  VectorParamsAs1DForOutWhenUnconnected=off
  Pitch (deg) : Outport  Port=2  VectorParamsAs1DForOutWhenUnconnected=off
  wires:
  wr/1 -> Sum/2, Sum1/1  "wr"
  0-inf/1 -> pu_elec->pu_mec/1
  pu_elec->pu_mec/1 -> Tracking Curve/1, Sum2/1, Switch/2  "Pmes"
  wref/1 -> Switch/1
  Switch/1 -> First-Order Filter1/1
  Sum1/1 -> Discrete PI Controller/1(Error)
  Constant2/1 -> Sum2/2  "Pref"
  Sum3/1 -> Rate Limiter   1/1
  Rate Limiter   1/1 -> "0-pitch_max "/1
  Gain2/1 -> 0-pitch_max/1
  Discrete PI Controller1/1(Out) -> Sum3/2  "Pitch_comp"
  Pmeas/1 -> 0-inf/1
  0-pitch_max/1 -> Sum3/1  "Pitch_contrl"
  "0-pitch_max "/1 -> First-Order Filter/1
  Sum/1 -> Gain2/1
  First-Order Filter/1 -> Pitch (deg)/1  "Pitch"
  Sum2/1 -> Discrete PI Controller1/1(Error)
  First-Order Filter1/1 -> Sum1/2, Sum/1  "wref"
  Tracking Curve/1 -> Switch/3
  Discrete PI Controller/1(Out) -> Sum4/1
  Sum4/1 -> Discrete PI Controller2/1(Error)
  IL/1 -> Sum4/2
  Discrete PI Controller2/1(Out) -> Duty_Cycle/1  "Duty cycle"

== system North_Country_Grid/Noble Clinton (Type 4, 100.5 MW)/Wind Farm/Control/Excitation Control system ==
  Flux : Inport
  wr : Inport  Port=2
  Discrete PI Controller : Subsystem  DialogController=POWERSYS.PowerSysDialog  mask(Discrete PI Controller){Kp=Kp_field, Ki=Ki_field, Par_Limits=[1 0]*Vf_limit, Init=init(9), Ts=Ts}
      mask prompts: Kp "Proportional gain (Kp):"; Ki "Integral gain (Ki):"; Par_Limits "Output limits: [ Upper   Lower ]"; Init "Output initial value:"; Ts "Sample time:"
      mask help: This block implements a discrete PI controller.
      mask init:
      | UpperLimit=Par_Limits(1);
      | LowerLimit=Par_Limits(2);
      | power_initmask();
      mask Help: This block is part of a subset of blocks in the Extras library that does not have documentation associated with it, other than the block mask description.
      mask Display: disp('PI');
  Divide : Product  Inputs=*/
  Flux_ref : Constant
  "Flux_ref " : Constant
  Sum4 : Sum  Inputs=|+-  InputSameDT=on  SaturateOnIntegerOverflow=on  OutDataTypeStr=Inherit: Same as first input
  Switch : Switch  Threshold=1  SaturateOnIntegerOverflow=off  InputSameDT=off
  avoid division by 0 : Saturate  UpperLimit=inf  LowerLimit=1e-6
  Vf : Outport  VectorParamsAs1DForOutWhenUnconnected=off
  wires:
  Sum4/1 -> Discrete PI Controller/1(Error)
  Discrete PI Controller/1(Out) -> Vf/1  "Vf"
  Flux/1 -> Sum4/2  "Flux"
  wr/1 -> Switch/2, avoid division by 0/1
  Flux_ref/1 -> Switch/3
  "Flux_ref "/1 -> Divide/1
  avoid division by 0/1 -> Divide/2
  Divide/1 -> Switch/1
  Switch/1 -> Sum4/1

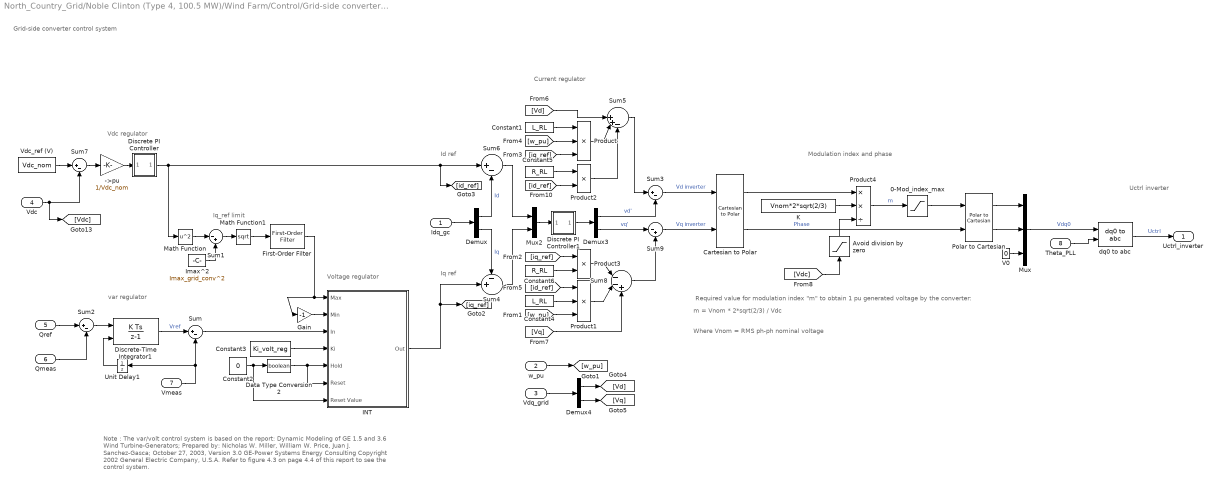
== system North_Country_Grid/Noble Clinton (Type 4, 100.5 MW)/Wind Farm/Control/Grid-side converter Control system ==
  note: Grid-side converter control system
  note: var regulator
  note: Voltage regulator
  note: Vdc regulator
  note: Iq_ref limit
  note: Current regulator
  note: Id ref
  note: Iq ref
  note: Required value for modulation index "m" to obtain 1 pu generated voltage by the converter:
  note: m = Vnom * 2*sqrt(2/3) / Vdc
  note: Where Vnom = RMS ph-ph nominal voltage
  note: Modulation index and phase
  note: Uctrl inverter
  note: Note :
      | The var/volt control system is based on the report:
      | Dynamic Modeling of GE 1.5 and 3.6 Wind Turbine-Generators;
      | Prepared by: Nicholas W. Miller, William W. Price, Juan J. Sanchez-Gasca;
      | October 27, 2003, Version 3.0
      | GE-Power Systems Energy Consulting
      | Copyright 2002 General Electric Company, U.S.A.
      |
      | Refer to figure 4.3 on page 4.4 of this report to see the control system.
  Idq_gc : Inport
  w_pu : Inport  Port=2
  Vdq_grid : Inport  Port=3
  Vdc : Inport  Port=4
  Qref : Inport  Port=5
  Qmeas : Inport  Port=6
  Vmeas : Inport  Port=7
  Theta_PLL : Inport  Port=8
  ->pu : Gain  Gain=1/Vdc_nom
  0-Mod_index_max : Saturate  UpperLimit=Mod_index_max  LowerLimit=0
  Avoid division by zero : Saturate  UpperLimit=1e6  LowerLimit=1e-6
  Cartesian to Polar : simulink_extras/Transformations/Cartesian to Polar
  Constant1 : Constant  Value=L_RL
  Constant2 : Constant  Value=0
  Constant3 : Constant  Value=Ki_volt_reg
  Constant4 : Constant  Value=L_RL
  Constant5 : Constant  Value=R_RL
  Constant6 : Constant  Value=R_RL
  Data Type Conversion2 : DataTypeConversion  OutDataTypeStr=boolean  SaturateOnIntegerOverflow=off  RndMeth=Floor
  Demux : Demux  Outputs=2
      settings: DisplayOption=none
  Demux3 : Demux  Outputs=2
      settings: DisplayOption=none
  Demux4 : Demux  Outputs=2
      settings: DisplayOption=none
  Discrete PI Controller : Subsystem  DialogController=POWERSYS.PowerSysDialog  mask(Discrete PI Controller){Kp=Kp_dc, Ki=Ki_dc, Par_Limits=[1 -1]*Imax_grid_conv, Init=0, Ts=Ts}
      mask prompts: Kp "Proportional gain (Kp):"; Ki "Integral gain (Ki):"; Par_Limits "Output limits: [ Upper   Lower ]"; Init "Output initial value:"; Ts "Sample time:"
      mask help: This block implements a discrete PI controller.
      mask init:
      | UpperLimit=Par_Limits(1);
      | LowerLimit=Par_Limits(2);
      | power_initmask();
      mask Help: This block is part of a subset of blocks in the Extras library that does not have documentation associated with it, other than the block mask description.
      mask Display: disp('PI');
  Discrete PI Controller1 : Subsystem  DialogController=POWERSYS.PowerSysDialog  mask(Discrete PI Controller){Kp=Kp_grid_side_cur_reg, Ki=Ki_grid_side_cur_reg, Par_Limits=[1 -1]*Current_reg_output_limit, Init=0, Ts=Ts}
      mask prompts: Kp "Proportional gain (Kp):"; Ki "Integral gain (Ki):"; Par_Limits "Output limits: [ Upper   Lower ]"; Init "Output initial value:"; Ts "Sample time:"
      mask help: This block implements a discrete PI controller.
      mask init:
      | UpperLimit=Par_Limits(1);
      | LowerLimit=Par_Limits(2);
      | power_initmask();
      mask Help: This block is part of a subset of blocks in the Extras library that does not have documentation associated with it, other than the block mask description.
      mask Display: disp('PI');
  Discrete-Time Integrator1 : DiscreteIntegrator  gainval=Ki_var_reg  InitialConditionSource=external  InitialCondition=1  SampleTime=Ts  LimitOutput=on  UpperSaturationLimit=Var_reg_output_hi_limit  LowerSaturationLimit=Var_reg_output_low_limit  ICPrevOutput=DiscIntNeverNeededParam  ICPrevScaledInput=DiscIntNeverNeededParam
  First-Order Filter : spsFirstOrderFilterLib/First-Order Filter  FilterType=Lowpass  Tc=Iq_ref_limit_time_constant  Ts=Ts  Initialize=on  Vac_Init=[0, 0, 0]  Vdc_Init=Imax_grid_conv  PlotResponse=off  FreqRange="[0,  200,  1]"
  Gain : Gain  Gain=-1  SaturateOnIntegerOverflow=on  OutDataTypeStr=Inherit: Same as input  ParamDataTypeStr=Inherit: Same as input
  INT : Subsystem  mask(Integrator  With  External  Dynamic  Limits (Discrete)){}
      mask Display: disp('Discrete-Time\n(Trapezoidal)\nIntegrator\n ')
  Imax^2 : Constant  Value=Imax_grid_conv^2
  K : Constant  Value=Vnom*2*sqrt(2/3)
  Math Function : Math  Operator=square  SignedPower=on
  Math Function1 : Math  Operator=sqrt  SignedPower=on
  Mux : Mux  Inputs=3
  Mux2 : Mux  Inputs=2
  Polar to Cartesian : simulink_extras/Transformations/Polar to Cartesian
  Product : Product  Inputs=3  InputSameDT=on  SaturateOnIntegerOverflow=on  OutDataTypeStr=Inherit: Same as first input
  Product1 : Product  Inputs=3  InputSameDT=on  SaturateOnIntegerOverflow=on  OutDataTypeStr=Inherit: Same as first input
  Product2 : Product  InputSameDT=on  SaturateOnIntegerOverflow=on  OutDataTypeStr=Inherit: Same as first input
  Product3 : Product  InputSameDT=on  SaturateOnIntegerOverflow=on  OutDataTypeStr=Inherit: Same as first input
  Product4 : Product  Inputs=**/  InputSameDT=on  SaturateOnIntegerOverflow=on  OutDataTypeStr=Inherit: Same as first input
  Sum{,2..3,6..7} (5 alike) : Sum  Inputs=|+-  InputSameDT=on  SaturateOnIntegerOverflow=on  OutDataTypeStr=Inherit: Same as first input
  Sum1 : Sum  Inputs=|-+  InputSameDT=on  SaturateOnIntegerOverflow=on  OutDataTypeStr=Inherit: Same as first input
  Sum4 : Sum  Inputs=-+|  InputSameDT=on  SaturateOnIntegerOverflow=on  OutDataTypeStr=Inherit: Same as first input
  Sum5 : Sum  Inputs=||++-  InputSameDT=on  SaturateOnIntegerOverflow=on  OutDataTypeStr=Inherit: Same as first input
  Sum8 : Sum  Inputs=|--+  InputSameDT=on  SaturateOnIntegerOverflow=on  OutDataTypeStr=Inherit: Same as first input
  Sum9 : Sum  Inputs=|-+  InputSameDT=on  SaturateOnIntegerOverflow=on  OutDataTypeStr=Inherit: Same as first input
  Unit Delay1 : UnitDelay  InitialCondition=1  SampleTime=Ts  HasFrameUpgradeWarning=on
  V0 : Constant  Value=0
  Vdc_ref (V) : Constant  Value=Vdc_nom
  dq0 to abc : spsdq0toabcLib/dq0 to abc  Alignment=90 degrees behind phase A axis
  Uctrl_inverter : Outport  VectorParamsAs1DForOutWhenUnconnected=off
  wires:
  Vdc/1 -> [Vdc], Sum7/2
  Vdq_grid/1 -> Demux4/1
  Sum7/1 -> ->pu/1
  ->pu/1 -> Discrete PI Controller/1(Error)
  Discrete PI Controller/1(Out) -> Math Function/1, [id_ref], Sum6/1
  Sum/1 -> INT/3(In)
  Constant2/1 -> Data Type Conversion2/1, INT/7(Reset Value)
  Data Type Conversion2/1 -> INT/5(Hold), INT/6(Reset)
  Gain/1 -> INT/2(Min)
  Constant3/1 -> INT/4(Ki)
  Discrete-Time Integrator1/1 -> Sum/1  "Vref"
  Vmeas/1 -> Unit Delay1/1, Sum/2
  Qmeas/1 -> Sum2/2
  Sum2/1 -> Discrete-Time Integrator1/1
  Unit Delay1/1 -> Discrete-Time Integrator1/2
  Math Function1/1 -> First-Order Filter/1
  Sum1/1 -> Math Function1/1
  Imax^2/1 -> Sum1/2
  Math Function/1 -> Sum1/1
  First-Order Filter/1 -> Gain/1, INT/1(Max)
  Constant4/1 -> Product1/2
  Discrete PI Controller1/1(Out) -> Demux3/1
  Mux2/1 -> Discrete PI Controller1/1(Error)
  Constant1/1 -> Product/1
  Demux/2 -> Sum4/1  "Iq"
  Demux/1 -> Sum6/2  "Id"
  Product/1 -> Sum5/2
  Constant5/1 -> Product2/1
  Constant6/1 -> Product3/2
  Product1/1 -> Sum8/2
  Product2/1 -> Sum5/3
  Product3/1 -> Sum8/1
  Sum6/1 -> Mux2/1
  Sum4/1 -> Mux2/2
  [w_pu] -> Product1/3
  [w_pu] -> Product/2
  [iq_ref] -> Product/3
  [id_ref] -> Product2/2
  [iq_ref] -> Product3/1
  [id_ref] -> Product1/1
  Demux3/1 -> Sum3/2  "vd'"
  Demux3/2 -> Sum9/1  "vq'"
  w_pu/1 -> [w_pu]
  Demux4/1 -> [Vd]
  Demux4/2 -> [Vq]
  [Vq] -> Sum8/3
  [Vd] -> Sum5/1
  Product4/1 -> 0-Mod_index_max/1  "m"
  K/1 -> Product4/2
  Avoid division by zero/1 -> Product4/3
  Cartesian to Polar/1 -> Product4/1
  [Vdc] -> Avoid division by zero/1
  Sum3/1 -> Cartesian to Polar/1  "Vd inverter"
  Sum9/1 -> Cartesian to Polar/2  "Vq inverter"
  Polar to Cartesian/2 -> Mux/2
  Polar to Cartesian/1 -> Mux/1
  V0/1 -> Mux/3
  Cartesian to Polar/2 -> Polar to Cartesian/2  "Phase"
  Mux/1 -> dq0 to abc/1  "Vdq0"
  dq0 to abc/1 -> Uctrl_inverter/1  "Uctrl"
  Idq_gc/1 -> Demux/1
  0-Mod_index_max/1 -> Polar to Cartesian/1
  Sum5/1 -> Sum3/1
  Sum8/1 -> Sum9/2
  Vdc_ref (V)/1 -> Sum7/1
  Qref/1 -> Sum2/1
  INT/1(Out) -> Sum4/2, [iq_ref]
  Theta_PLL/1 -> dq0 to abc/2
